simulink model "WindSpeed"  (R2024a)
settings: Solver=FixedStepAuto  StartTime=0.0  StopTime=inf  RelTol=1e-3
undefined symbols (not defined in the file or in its folder): DiscIntNeverNeededParam
libraries: simulink x5, dspfdesign x2
settings Model: Creator=12650018  LastModifiedBy=glazzerini
settings SolverCC: AlgebraicLoopSolver=TrustRegion
settings DebuggingCC: UnconnectedInputMsg=warning  UnconnectedOutputMsg=warning  UnconnectedLineMsg=warning
settings ModelReferenceCC: EnableRefExpFcnMdlSchedulingChecks=on
settings RTWCC: GPUComputeCapability=3.5

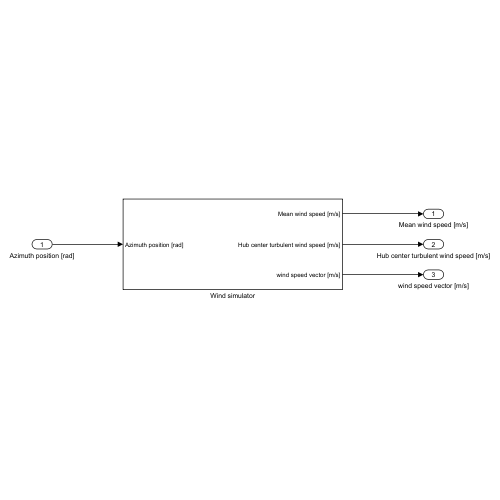
[thumbnail: Simulink's stored preview of the top-level diagram]
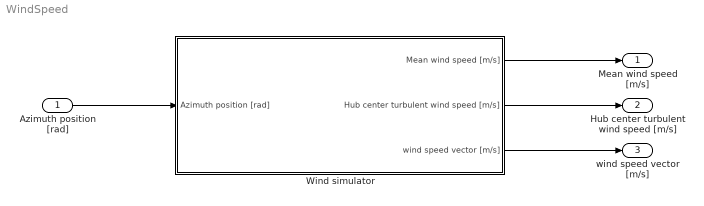
== system WindSpeed ==
  Azimuth position [rad] : Inport
  Wind simulator : Subsystem  mask(Wind speed field simulator){Ts=0.01, SimCase=5, WindSpdMean=11, Seed=12, ScaleTurbulence=1, WindShearVert=0, EnableTurbulence=1, SineAmplitude=0.1, SineFrequency=0.1, RampSlope=0.003, ECDmaxWind=0, SpeedSlope=0, ECDTime=0, ECDduration=1, ECDfinalYaw=0, R_eq=120, twrHeight=150}
      mask prompts: Ts "Sampling time [s]"; SimCase "Type of wind speed"; WindSpdMean "Mean wind speed [m/s]"; Seed "Initial turbulence seed [-]"; ScaleTurbulence "Turbulence gain [-]"; WindShearVert "Vertical wind shear exponential [-]"; EnableTurbulence "Enable turbulences [0,1]"; SineAmplitude "Amplitude of sine wind speed [m/s]"; SineFrequency "Frequency of sinusoidal wind speed [rad/s]"; RampSlope "Ramp slope [m/s2]"; ECDmaxWind "Maximum gust amplitude [m/s]"; SpeedSlope "Gust increase rate [m/s2]"; ECDTime "Gust triggering time [s]"; ECDduration "ECD maximum time duration [s]"; ECDfinalYaw "Yaw missalignment at ECD end [rad]"; R_eq "Rotor radius [m]"; twrHeight "Tower height [m]"
      mask help:
      | Wind speed simulator. Set the simulation to the desired wind case:
      | 1. Constant 5 m/s wind speed
      | 2. Constant 9 m/s wind speed
      | 3. Constant 15 m/s wind speed
      | 4. Wind speed ramp
      | 5. Wind speed sine
      | 6. ECD event
      | 7. User defined wind (wind speed defined by parameter).
      mask Help: EIC SEWPG 2024.
      mask DialogControl Container3 Prompt: Wind parameters
      mask DialogControl Turbulences Prompt: Turbulence parameters
      mask DialogControl Sinusoidalwind Prompt: Sinusoidal wind
      mask DialogControl Container7 Prompt: Ramp Wind
      mask DialogControl Container9 Prompt: ECD wind
      mask DialogControl Container4 Prompt: Turbine parameters
  Mean wind speed [m/s] : Outport
  Hub center turbulent wind speed [m/s] : Outport  Port=2
  wind speed vector [m/s] : Outport  Port=3
  wires:
  Azimuth position [rad]/1 -> Wind simulator/1(Azimuth position [rad])
  Wind simulator/1(Mean wind speed [m/s]) -> Mean wind speed [m/s]/1
  Wind simulator/2(Hub center turbulent wind speed [m/s]) -> Hub center turbulent wind speed [m/s]/1
  Wind simulator/3(wind speed vector [m/s]) -> wind speed vector [m/s]/1

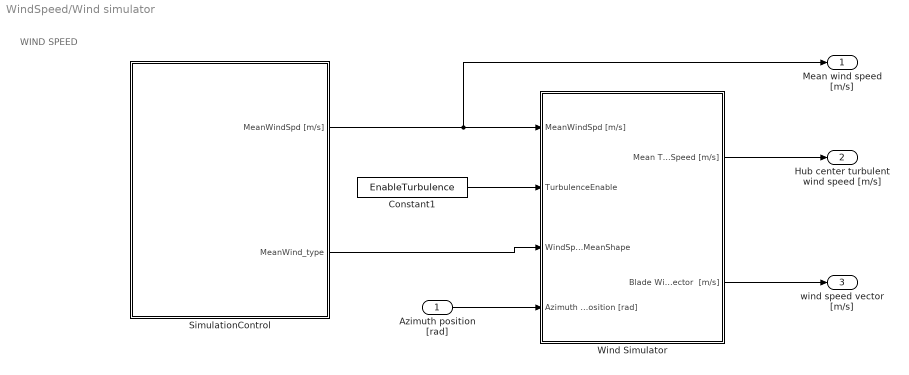
== system WindSpeed/Wind simulator ==
  note: WIND SPEED
  Azimuth position [rad] : Inport
  Constant1 : Constant  Value=EnableTurbulence
  SimulationControl : Subsystem
  Wind Simulator : Subsystem
  Mean wind speed [m/s] : Outport
  Hub center turbulent wind speed [m/s] : Outport  Port=2
  wind speed vector [m/s] : Outport  Port=3
  wires:
  SimulationControl/2(MeanWind_type) -> Wind Simulator/3(WindSpeedMeanShape)
  SimulationControl/1(MeanWindSpd [m/s]) -> Mean wind speed [m/s]/1, Wind Simulator/1(MeanWindSpd [m/s])
  Constant1/1 -> Wind Simulator/2(TurbulenceEnable)
  Wind Simulator/1(Mean Turbulent Wind Speed [m/s]) -> Hub center turbulent wind speed [m/s]/1
  Azimuth position [rad]/1 -> Wind Simulator/4(Azimuth position [rad])
  Wind Simulator/2(Blade Wind Speed Vector  [m/s]) -> wind speed vector [m/s]/1

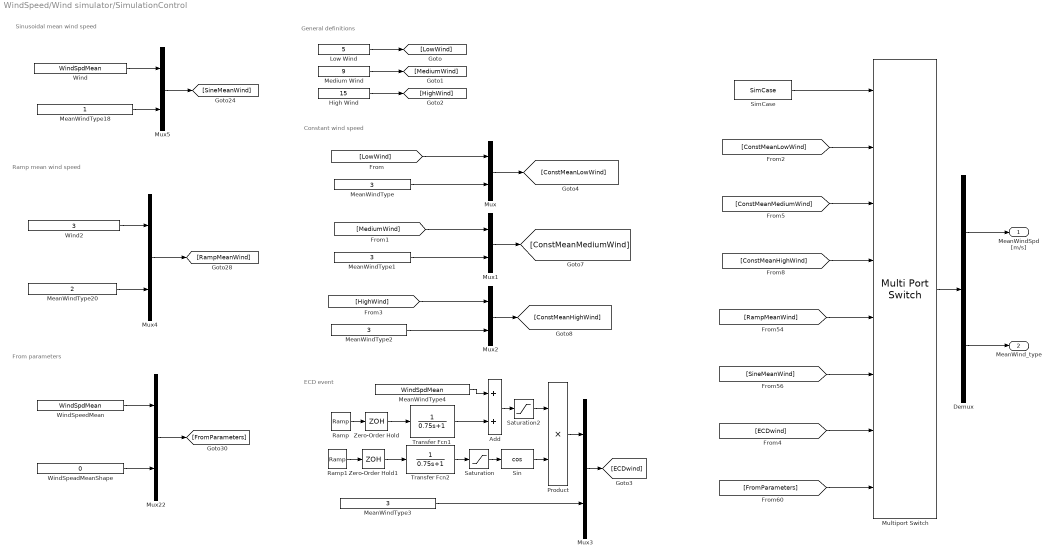
== system WindSpeed/Wind simulator/SimulationControl ==
  note: From parameters
  note: Sinusoidal mean wind speed
  note: General definitions
  note: Constant wind speed
  note: Ramp mean wind speed
  note: ECD event
  Add : Sum
  Demux : Demux  Outputs=2
  High Wind : Constant  Value=15
  Low Wind : Constant  Value=5
  MeanWindType{,1..3} (4 alike) : Constant  Value=3
  MeanWindType18 : Constant
  MeanWindType20 : Constant  Value=2
  MeanWindType4 : Constant  Value=WindSpdMean
  Medium Wind : Constant  Value=9
  Multiport Switch : MultiPortSwitch  Inputs=7  SaturateOnIntegerOverflow=off  InputSameDT=off
  Mux{,1..5,22} (7 alike) : Mux  Inputs=2
  Product : Product
  Ramp : simulink/Sources/Ramp  slope=SpeedSlope  start=ECDTime  InitialOutput=0
  Ramp1 : simulink/Sources/Ramp  slope=ECDfinalYaw/ECDduration  start=ECDTime  InitialOutput=0
  Saturation : Saturate  UpperLimit=ECDfinalYaw  LowerLimit=-ECDfinalYaw
  Saturation2 : Saturate  UpperLimit=ECDmaxWind  LowerLimit=0
  SimCase : Constant  Value=SimCase
  Sin : Trigonometry  Operator=cos
  Transfer Fcn1 : TransferFcn  Denominator=[0.75 1]
  Transfer Fcn2 : TransferFcn  Denominator=[0.75 1]
  Wind : Constant  Value=WindSpdMean
  Wind2 : Constant  Value=3
  WindSpeadMeanShape : Constant  Value=0
  WindSpeedMean : Constant  Value=WindSpdMean
  Zero-Order Hold : ZeroOrderHold  SampleTime=Ts
  Zero-Order Hold1 : ZeroOrderHold  SampleTime=Ts
  MeanWindSpd [m/s] : Outport
  MeanWind_type : Outport  Port=2
  wires:
  WindSpeadMeanShape/1 -> Mux22/2
  MeanWindType20/1 -> Mux4/2
  MeanWindType18/1 -> Mux5/2
  [HighWind] -> Mux2/1
  Mux2/1 -> [ConstMeanHighWind]
  MeanWindType2/1 -> Mux2/2
  MeanWindType1/1 -> Mux1/2
  [MediumWind] -> Mux1/1
  Mux1/1 -> [ConstMeanMediumWind]
  MeanWindType/1 -> Mux/2
  Demux/2 -> MeanWind_type/1
  [ConstMeanLowWind] -> Multiport Switch/2
  [ConstMeanMediumWind] -> Multiport Switch/3
  [ConstMeanHighWind] -> Multiport Switch/4
  [RampMeanWind] -> Multiport Switch/5
  [SineMeanWind] -> Multiport Switch/6
  SimCase/1 -> Multiport Switch/1
  Demux/1 -> MeanWindSpd [m/s]/1
  Mux22/1 -> [FromParameters]
  Mux4/1 -> [RampMeanWind]
  Mux5/1 -> [SineMeanWind]
  Mux/1 -> [ConstMeanLowWind]
  [LowWind] -> Mux/1
  High Wind/1 -> [HighWind]
  Medium Wind/1 -> [MediumWind]
  Low Wind/1 -> [LowWind]
  Multiport Switch/1 -> Demux/1
  Wind/1 -> Mux5/1
  Wind2/1 -> Mux4/1
  WindSpeedMean/1 -> Mux22/1
  Mux3/1 -> [ECDwind]
  Zero-Order Hold1/1 -> Transfer Fcn2/1
  Ramp/1 -> Zero-Order Hold/1
  Product/1 -> Mux3/1
  MeanWindType3/1 -> Mux3/2
  Transfer Fcn2/1 -> Saturation/1
  Sin/1 -> Product/2
  Zero-Order Hold/1 -> Transfer Fcn1/1
  Ramp1/1 -> Zero-Order Hold1/1
  [ECDwind] -> Multiport Switch/7
  [FromParameters] -> Multiport Switch/8
  Saturation/1 -> Sin/1
  Add/1 -> Saturation2/1
  MeanWindType4/1 -> Add/1
  Transfer Fcn1/1 -> Add/2
  Saturation2/1 -> Product/1

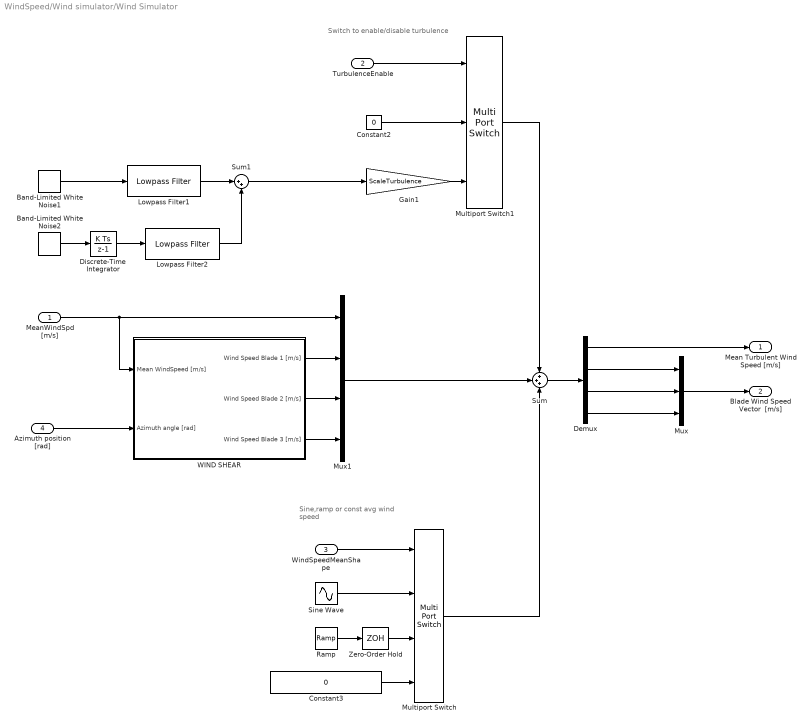
== system WindSpeed/Wind simulator/Wind Simulator ==
  note: Switch to enable/disable turbulence
  note: Sine,ramp or const
      |  avg wind speed
  MeanWindSpd [m/s] : Inport
  TurbulenceEnable : Inport  Port=2
  WindSpeedMeanShape : Inport  Port=3
  Azimuth position [rad] : Inport  Port=4
  Band-Limited White Noise1 : simulink/Sources/Band-Limited White Noise  Cov=[0.03]  Ts=Ts  seed=Seed+1337
  Band-Limited White Noise2 : simulink/Sources/Band-Limited White Noise  Cov=[1]  Ts=Ts  seed=Seed
  Constant2 : Constant  Value=0  SampleTime=-1
  Constant3 : Constant  Value=0  SampleTime=-1
  Demux : Demux
  Discrete-Time Integrator : DiscreteIntegrator  gainval=0.15  SampleTime=Ts  ICPrevOutput=DiscIntNeverNeededParam  ICPrevScaledInput=DiscIntNeverNeededParam
  Gain1 : Gain  Gain=ScaleTurbulence
  Lowpass Filter1 : dspfdesign/Lowpass Filter  FilterType=FIR  DesignForMinimumOrder=on  FilterOrder=50  PassbandFrequency=1e-3  StopbandFrequency=1e-1  PassbandRipple=0.1  StopbandAttenuation=80  SampleRateMode=Specify on dialog  SampleRate=1/Ts  SimulateUsing=Interpreted execution  roundingMode=Floor  coeffsDataTypeStr=fixdt(1,16)
  Lowpass Filter2 : dspfdesign/Lowpass Filter  FilterType=FIR  DesignForMinimumOrder=on  FilterOrder=50  PassbandFrequency=1e-3  StopbandFrequency=1e-1  PassbandRipple=0.1  StopbandAttenuation=80  SampleRateMode=Specify on dialog  SampleRate=1/Ts  SimulateUsing=Interpreted execution  roundingMode=Floor  coeffsDataTypeStr=fixdt(1,16)
  Multiport Switch : MultiPortSwitch  SaturateOnIntegerOverflow=off  InputSameDT=off
  Multiport Switch1 : MultiPortSwitch  DataPortOrder=Zero-based contiguous  Inputs=2  zeroidx=on  SaturateOnIntegerOverflow=off  InputSameDT=off
  Mux : Mux  Inputs=3
  Mux1 : Mux
  Ramp : simulink/Sources/Ramp  slope=RampSlope  start=0  InitialOutput=0
  Sine Wave : Sin  Amplitude=SineAmplitude  Frequency=SineFrequency  Phase=deg2rad(0)  SampleTime=Ts
  Sum : Sum  Inputs=+++
  Sum1 : Sum  Inputs=|++
  WIND SHEAR : Subsystem
  Zero-Order Hold : ZeroOrderHold  SampleTime=Ts
  Mean Turbulent Wind Speed [m/s] : Outport
  Blade Wind Speed Vector  [m/s] : Outport  Port=2
  wires:
  Zero-Order Hold/1 -> Multiport Switch/3
  Ramp/1 -> Zero-Order Hold/1
  Sum1/1 -> Gain1/1
  Discrete-Time Integrator/1 -> Lowpass Filter2/1
  Lowpass Filter2/1 -> Sum1/2
  Band-Limited White Noise2/1 -> Discrete-Time Integrator/1
  TurbulenceEnable/1 -> Multiport Switch1/1
  Multiport Switch/1 -> Sum/3
  WindSpeedMeanShape/1 -> Multiport Switch/1
  Constant3/1 -> Multiport Switch/4
  Sine Wave/1 -> Multiport Switch/2
  Constant2/1 -> Multiport Switch1/2
  Multiport Switch1/1 -> Sum/1
  Mux1/1 -> Sum/2
  Gain1/1 -> Multiport Switch1/3
  Mux/1 -> Blade Wind Speed Vector  [m/s]/1
  Azimuth position [rad]/1 -> WIND SHEAR/2(Azimuth angle [rad])
  WIND SHEAR/3(Wind Speed Blade 3 [m/s]) -> Mux1/4
  WIND SHEAR/2(Wind Speed Blade 2 [m/s]) -> Mux1/3
  WIND SHEAR/1(Wind Speed Blade 1 [m/s]) -> Mux1/2
  MeanWindSpd [m/s]/1 -> WIND SHEAR/1(Mean WindSpeed [m/s]), Mux1/1
  Sum/1 -> Demux/1
  Demux/1 -> Mean Turbulent Wind Speed [m/s]/1
  Demux/2 -> Mux/1
  Demux/3 -> Mux/2
  Demux/4 -> Mux/3
  Lowpass Filter1/1 -> Sum1/1
  Band-Limited White Noise1/1 -> Lowpass Filter1/1

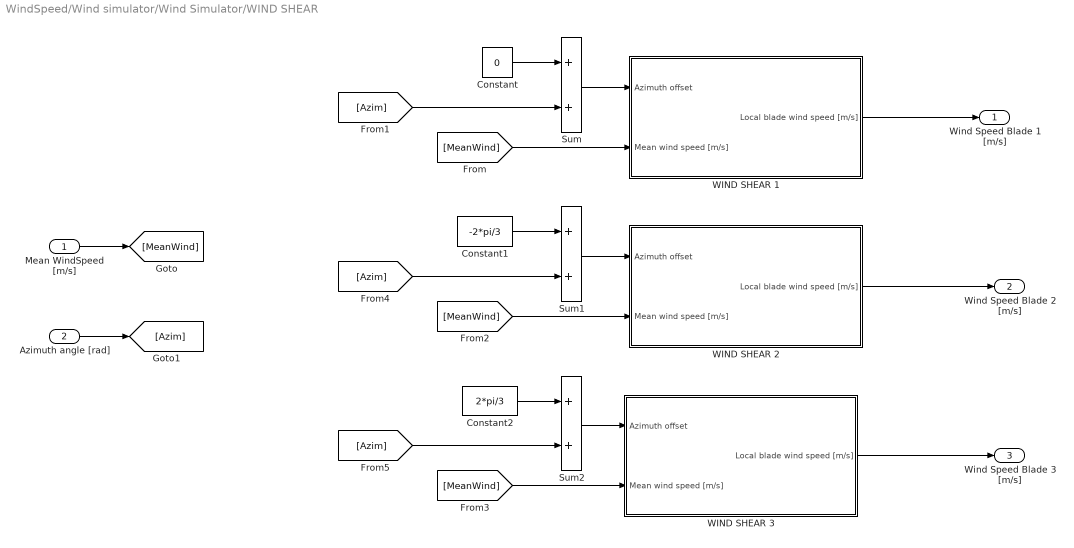
== system WindSpeed/Wind simulator/Wind Simulator/WIND SHEAR ==
  Mean WindSpeed [m/s] : Inport
  Azimuth angle [rad] : Inport  Port=2
  Constant : Constant  Value=0
  Constant1 : Constant  Value=-2*pi/3
  Constant2 : Constant  Value=2*pi/3
  Sum : Sum
  Sum1 : Sum
  Sum2 : Sum
  WIND SHEAR 1 : Subsystem
  WIND SHEAR 2 : Subsystem
  WIND SHEAR 3 : Subsystem
  Wind Speed Blade 1 [m/s] : Outport
  Wind Speed Blade 2 [m/s] : Outport  Port=2
  Wind Speed Blade 3 [m/s] : Outport  Port=3
  wires:
  Mean WindSpeed [m/s]/1 -> [MeanWind]
  Azimuth angle [rad]/1 -> [Azim]
  WIND SHEAR 1/1(Local blade wind speed [m/s]) -> Wind Speed Blade 1 [m/s]/1
  WIND SHEAR 2/1(Local blade wind speed [m/s]) -> Wind Speed Blade 2 [m/s]/1
  WIND SHEAR 3/1(Local blade wind speed [m/s]) -> Wind Speed Blade 3 [m/s]/1
  [MeanWind] -> WIND SHEAR 1/2(Mean wind speed [m/s])
  [MeanWind] -> WIND SHEAR 2/2(Mean wind speed [m/s])
  [MeanWind] -> WIND SHEAR 3/2(Mean wind speed [m/s])
  Sum/1 -> WIND SHEAR 1/1(Azimuth offset)
  [Azim] -> Sum/2
  [Azim] -> Sum1/2
  Sum1/1 -> WIND SHEAR 2/1(Azimuth offset)
  [Azim] -> Sum2/2
  Sum2/1 -> WIND SHEAR 3/1(Azimuth offset)
  Constant/1 -> Sum/1
  Constant1/1 -> Sum1/1
  Constant2/1 -> Sum2/1

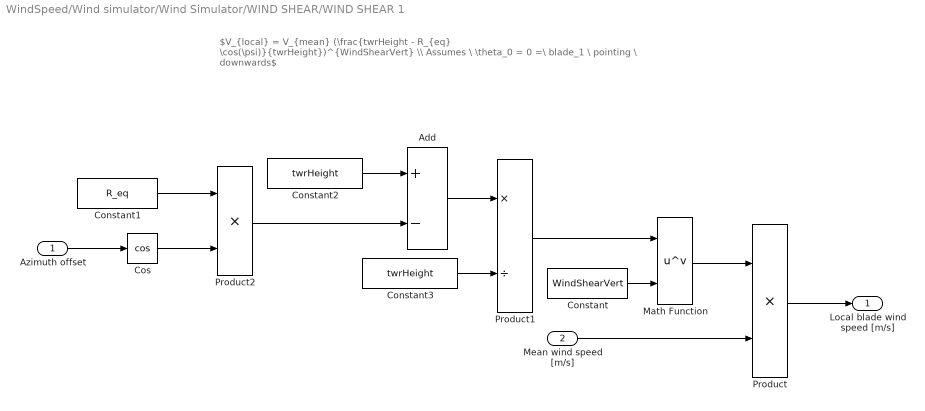
== system WindSpeed/Wind simulator/Wind Simulator/WIND SHEAR/WIND SHEAR 1 ==
  note: $V_{local} = V_{mean} (\frac{twrHeight - R_{eq} \cos(\psi)}{twrHeight})^{WindShearVert} \\ Assumes \ \theta_0 = 0 =\ blade_1 \ pointing \ downwards$
  Azimuth offset : Inport
  Mean wind speed [m/s] : Inport  Port=2
  Add : Sum  Inputs=+-
  Constant : Constant  Value=WindShearVert
  Constant1 : Constant  Value=R_eq
  Constant2 : Constant  Value=twrHeight
  Constant3 : Constant  Value=twrHeight
  Cos : Trigonometry  Operator=cos
  Math Function : Math  Operator=pow
  Product : Product
  Product1 : Product  Inputs=*/
  Product2 : Product  Inputs=**
  Local blade wind speed [m/s] : Outport
  wires:
  Cos/1 -> Product2/2
  Product2/1 -> Add/2
  Constant3/1 -> Product1/2
  Constant2/1 -> Add/1
  Constant1/1 -> Product2/1
  Mean wind speed [m/s]/1 -> Product/2
  Constant/1 -> Math Function/2
  Add/1 -> Product1/1
  Math Function/1 -> Product/1
  Product1/1 -> Math Function/1
  Azimuth offset/1 -> Cos/1
  Product/1 -> Local blade wind speed [m/s]/1

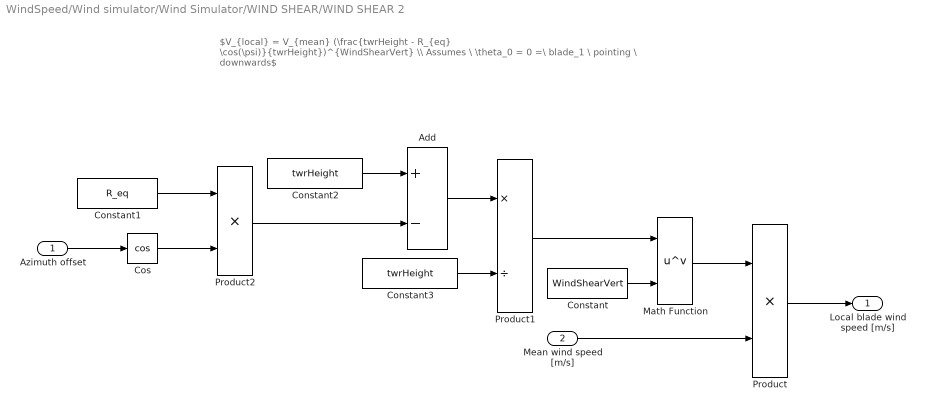
== system WindSpeed/Wind simulator/Wind Simulator/WIND SHEAR/WIND SHEAR 2 ==
  note: $V_{local} = V_{mean} (\frac{twrHeight - R_{eq} \cos(\psi)}{twrHeight})^{WindShearVert} \\ Assumes \ \theta_0 = 0 =\ blade_1 \ pointing \ downwards$
  Azimuth offset : Inport
  Mean wind speed [m/s] : Inport  Port=2
  Add : Sum  Inputs=+-
  Constant : Constant  Value=WindShearVert
  Constant1 : Constant  Value=R_eq
  Constant2 : Constant  Value=twrHeight
  Constant3 : Constant  Value=twrHeight
  Cos : Trigonometry  Operator=cos
  Math Function : Math  Operator=pow
  Product : Product
  Product1 : Product  Inputs=*/
  Product2 : Product  Inputs=**
  Local blade wind speed [m/s] : Outport
  wires:
  Product/1 -> Local blade wind speed [m/s]/1
  Azimuth offset/1 -> Cos/1
  Product1/1 -> Math Function/1
  Math Function/1 -> Product/1
  Add/1 -> Product1/1
  Constant/1 -> Math Function/2
  Mean wind speed [m/s]/1 -> Product/2
  Constant1/1 -> Product2/1
  Constant2/1 -> Add/1
  Constant3/1 -> Product1/2
  Product2/1 -> Add/2
  Cos/1 -> Product2/2

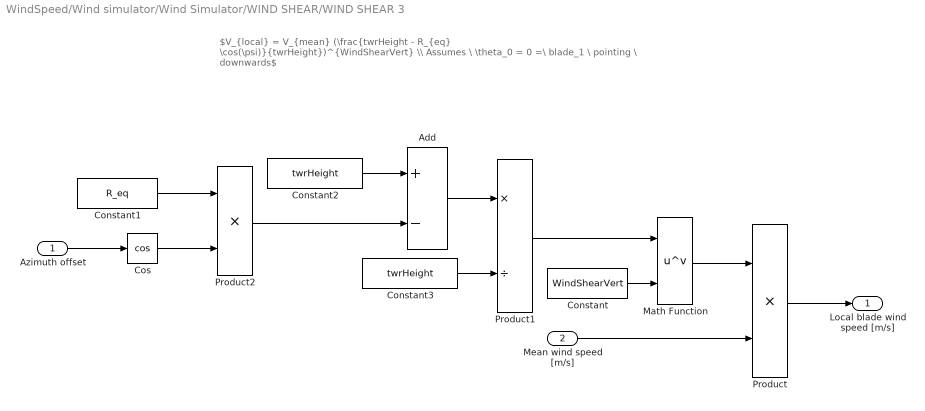
== system WindSpeed/Wind simulator/Wind Simulator/WIND SHEAR/WIND SHEAR 3 ==
  note: $V_{local} = V_{mean} (\frac{twrHeight - R_{eq} \cos(\psi)}{twrHeight})^{WindShearVert} \\ Assumes \ \theta_0 = 0 =\ blade_1 \ pointing \ downwards$
  Azimuth offset : Inport
  Mean wind speed [m/s] : Inport  Port=2
  Add : Sum  Inputs=+-
  Constant : Constant  Value=WindShearVert
  Constant1 : Constant  Value=R_eq
  Constant2 : Constant  Value=twrHeight
  Constant3 : Constant  Value=twrHeight
  Cos : Trigonometry  Operator=cos
  Math Function : Math  Operator=pow
  Product : Product
  Product1 : Product  Inputs=*/
  Product2 : Product  Inputs=**
  Local blade wind speed [m/s] : Outport
  wires:
  Cos/1 -> Product2/2
  Product2/1 -> Add/2
  Constant3/1 -> Product1/2
  Constant2/1 -> Add/1
  Constant1/1 -> Product2/1
  Mean wind speed [m/s]/1 -> Product/2
  Constant/1 -> Math Function/2
  Add/1 -> Product1/1
  Math Function/1 -> Product/1
  Product1/1 -> Math Function/1
  Azimuth offset/1 -> Cos/1
  Product/1 -> Local blade wind speed [m/s]/1
